simulink model "task_1"  (R2023a)
settings: Solver=VariableStepAuto  StartTime=0.0  StopTime=5.0  RelTol=1e-8
settings Model: Creator=user  LastModifiedBy=user

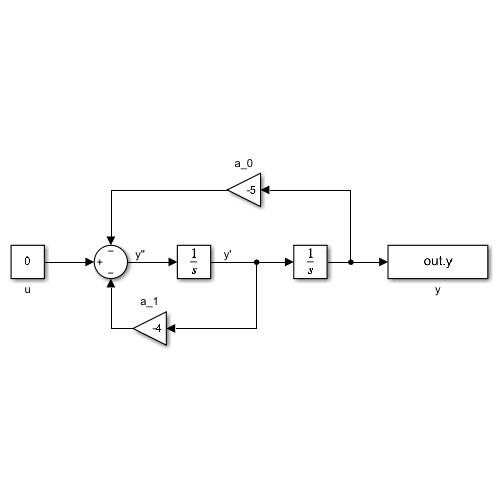
[thumbnail: Simulink's stored preview of the top-level diagram]
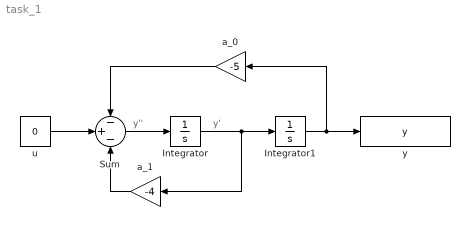
== system task_1 ==
  note: y'
  note: y''
  Integrator : Integrator  InitialCondition=1
  Integrator1 : Integrator  InitialCondition=1
  Sum : Sum  Inputs=-+-
  a_0 : Gain  Gain=-5
  a_1 : Gain  Gain=-4
  u : Constant  Value=0
  y : ToWorkspace  VariableName=y  SaveFormat=Timeseries  SampleTime=-1
  wires:
  Sum/1 -> Integrator/1
  u/1 -> Sum/2
  Integrator/1 -> a_1/1, Integrator1/1
  Integrator1/1 -> a_0/1, y/1
  a_0/1 -> Sum/1
  a_1/1 -> Sum/3
